simulink model "workshopMatlabCode"  (R2023a)
settings: Solver=VariableStepAuto  StartTime=0.0  StopTime=10.0  RelTol=1e-3
libraries: dspsrcs4 x2
settings Model: Creator=Ditte  LastModifiedBy=Ditte

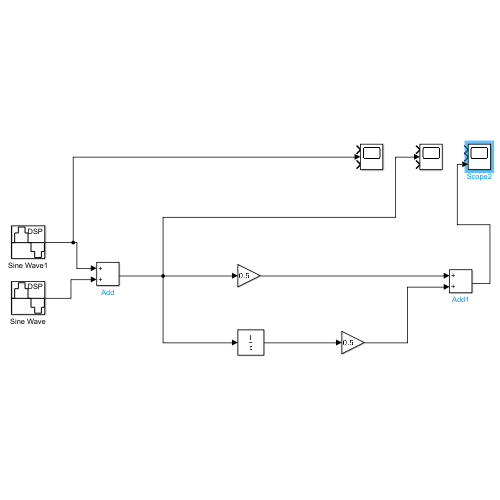
[thumbnail: Simulink's stored preview of the top-level diagram]
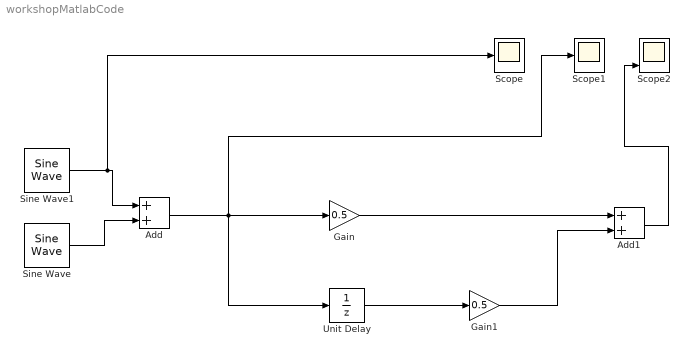
== system workshopMatlabCode ==
  Add : Sum
  Add1 : Sum
  Gain : Gain  Gain=0.5
  Gain1 : Gain  Gain=0.5
  Scope : Scope  NumInputPorts=3
  Scope1 : Scope  NumInputPorts=3
  Scope2 : Scope  NumInputPorts=3
  Sine Wave : dspsrcs4/Sine Wave  Amplitude=2.5  Frequency=2.8647889789  Phase=0  SampleMode=Discrete  OutComplex=Real  CompMethod=Trigonometric fcn  TableSize=Speed  SampleTime=0.2  SamplesPerFrame=1  ResetState=Restart at time zero  OutputFrames=off  dataType=double  wordLen=16  udDataType=sfix(16)  fracBitsMode=Best precision  numFracBits=15  OutDataTypeStr=double  LastOutDataTypeStr=double
  Sine Wave1 : dspsrcs4/Sine Wave  Amplitude=10  Frequency=0.1591549433  Phase=0  SampleMode=Discrete  OutComplex=Real  CompMethod=Trigonometric fcn  TableSize=Speed  SampleTime=0.2  SamplesPerFrame=1  ResetState=Restart at time zero  OutputFrames=off  dataType=double  wordLen=16  udDataType=sfix(16)  fracBitsMode=Best precision  numFracBits=15  OutDataTypeStr=double  LastOutDataTypeStr=double
  Unit Delay : UnitDelay  SampleTime=-1  HasFrameUpgradeWarning=on
  wires:
  Sine Wave/1 -> Add/2
  Sine Wave1/1 -> Scope/2, Add/1
  Add/1 -> Scope1/2, Unit Delay/1, Gain/1
  Unit Delay/1 -> Gain1/1
  Gain/1 -> Add1/1
  Gain1/1 -> Add1/2
  Add1/1 -> Scope2/3
